simulink model "practice4"  (Simulink 7.9)
settings: Solver=ode45  StartTime=0.0  StopTime=40  RelTol=1e-3
libraries: simulink x1
settings Model: Creator=sony  LastModifiedBy=sony

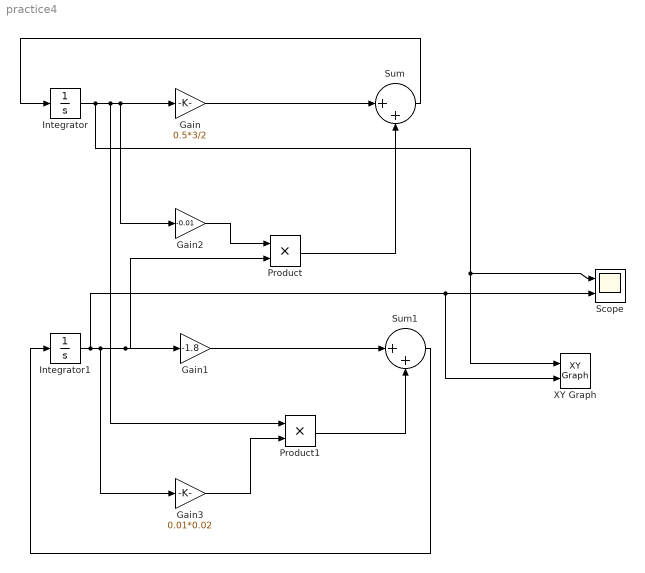
== system practice4 ==
  Gain : Gain  Gain=0.5*3/2
  Gain1 : Gain  Gain=-1.8
  Gain2 : Gain  Gain=-0.01
  Gain3 : Gain  Gain=0.01*0.02
  Integrator : Integrator  InitialCondition=140000
  Integrator1 : Integrator  InitialCondition=10
  Product : Product  RndMeth=Zero
  Product1 : Product  RndMeth=Zero
  Scope : Scope  NumInputPorts=2
      settings: YMin=-5~-5  YMax=5~5
  Sum : Sum  Inputs=|++
  Sum1 : Sum  Inputs=|++
  XY Graph : simulink/Sinks/XY Graph  xmin=0  xmax=160000  ymin=0  ymax=5000  st=-1
  wires:
  Integrator/1 -> Gain/1, Gain2/1, Product1/1, Scope/1, XY Graph/1
  Integrator1/1 -> Product/2, Gain1/1, Gain3/1, Scope/2, XY Graph/2
  Gain2/1 -> Product/1
  Gain/1 -> Sum/1
  Product/1 -> Sum/2
  Gain3/1 -> Product1/2
  Gain1/1 -> Sum1/1
  Product1/1 -> Sum1/2
  Sum/1 -> Integrator/1
  Sum1/1 -> Integrator1/1
